simulink model "Simscape_Benchmark_SIM1"  (R2021a)
settings: Solver=ode45  StartTime=0.0  StopTime=PHASE.Ttotal  FixedStep=Benchmark.Sim.Tint  RelTol=1e-5  AbsTol=1e-6
undefined symbols (not defined in the file): Actuators, Analysis, antisym, Benchmark, Bus, Disturbance, FSM, IntialCond, ISOL, K_Coarse_disc_t, Kslew_opt_disc_zoh, Model, MPS, PAYLOAD, PHASE, PMA, RWIsol, RWS, SA, Sensors, Slew, slosh, thr, X, Y, Z
libraries: sm_lib x215, nesl_utility x148, simulink x65, cstblocks x36, sharedtransform x4, vrlib x3, RCTblocks x1
(part 2 of 9)

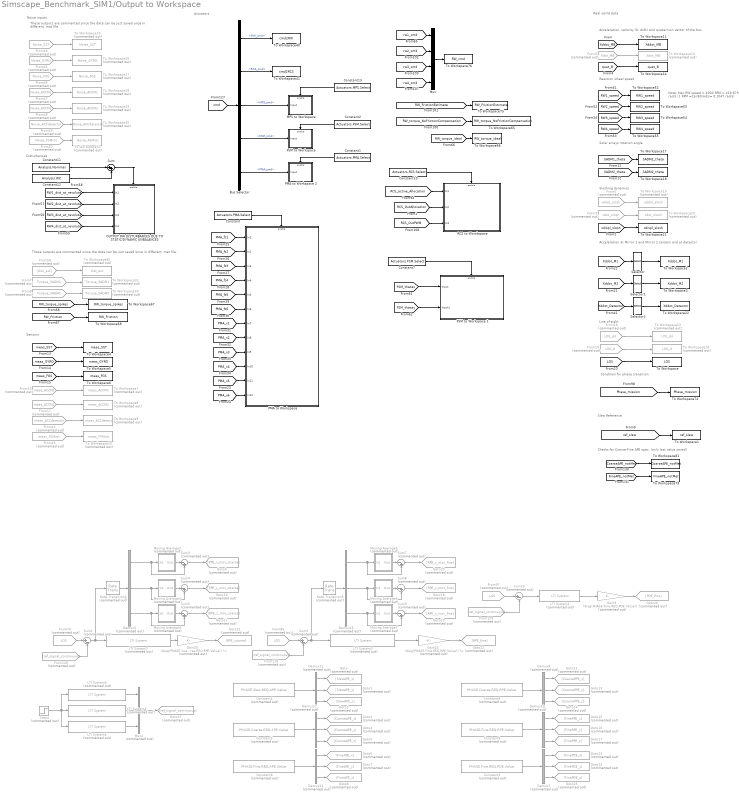
== system Simscape_Benchmark_SIM1/Output to Workspace ==
  note: Note:
      | Max RW speed = 4000 RPM = 418.879 rad/s
      |
      | (1 RPM =2pi/60rad/s= 0.1047 rad/s)
  note: Disturbances
  note: Actuators
  note: Noise inputs
  note: Real world data
  note: Sensors
  note: These outputs are commented since the data can be just saved once in different .mat file.
  note: These outputs are commented since the data can be just saved once in different .mat file.
  note: Acceleration, velocity (6- dofs) and quaternion vector of the bus
  note: Reaction wheel speed
  note: Solar arrays rotation angle
  note: Sloshing dynamics
  note: Acceleration at Mirror 1 and Mirror 2 centers and at detector
  note: Line of sight
  note: Condition for phase transition
  note: Checks for Coarse-Fine APE spec. (only last value saved)
  note: Slew Reference
  Bus Selector : BusSelector  OutputSignals=RW_cmd,RCS_cmd,MPS_cmd,FSM_cmd,PMA_cmd
  Constant : Constant  Value=Actuators.PMA.Select
  Constant1 : Constant  Value=Actuators.PMA.Select
  Constant10 : Constant  Value=Actuators.RCS.Select
  Constant11 : Constant  Value=Analysis.Nominal
  Constant12 : Constant  Value=Analysis.WC
  Constant13 : Constant  Value=Actuators.MPS.Select
  Constant2 : Constant  Value=Actuators.FSM.Select
  Constant3 : Constant  Commented=on  Value=PHASE.Fine.REQ.PDE.Value
  Constant4 : Constant  Commented=on  Value=PHASE.Slew.REQ.APE.Value
  Constant5 : Constant  Commented=on  Value=PHASE.Coarse.REQ.APE.Value
  Constant6 : Constant  Commented=on  Value=PHASE.Fine.REQ.APE.Value
  Constant7 : Constant  Value=Actuators.FSM.Select
  Constant8 : Constant  Commented=on  Value=PHASE.Coarse.REQ.RPE.Value
  Constant9 : Constant  Commented=on  Value=PHASE.Fine.REQ.RPE.Value
  Demux{3,7,9..13,15} (8 alike) : Demux  Commented=on  Outputs=3
  FSM to Workspace : Subsystem  TreatAsAtomicUnit=on
  FSM to Workspace 1 : Subsystem  TreatAsAtomicUnit=on
  From116 : From  Commented=on  GotoTag=ref_signal_continuous
  From120 : From  Commented=on  GotoTag=ref_signal_continuous
  From128 : From  Commented=on  GotoTag=ref_signal_continuous
  From16 : From  Commented=on  GotoTag=meas_ACCM1  TagVisibility=global
  From17 : From  Commented=on  GotoTag=meas_ACCM2  TagVisibility=global
  From18 : From  Commented=on  GotoTag=LOS_dd  TagVisibility=global
  From19 : From  Commented=on  GotoTag=LOS_d  TagVisibility=global
  From3 : From  Commented=on  GotoTag=xdot_slosh  TagVisibility=global
  From42 : From  Commented=on  GotoTag=meas_ACCdetector  TagVisibility=global
  From43 : From  Commented=on  GotoTag=meas_FSMrot  TagVisibility=global
  From44 : From  Commented=on  GotoTag=Noise_SST  TagVisibility=global
  From45 : From  Commented=on  GotoTag=Noise_GYRO  TagVisibility=global
  From46 : From  Commented=on  GotoTag=Noise_FGS  TagVisibility=global
  From47 : From  Commented=on  GotoTag=Noise_ACCM1  TagVisibility=global
  From48 : From  Commented=on  GotoTag=Noise_ACCM2  TagVisibility=global
  From49 : From  Commented=on  GotoTag=Noise_ACCdetector  TagVisibility=global
  From5 : From  Commented=on  GotoTag=xddot_slosh  TagVisibility=global
  From50 : From  Commented=on  GotoTag=Noise_FSMrot  TagVisibility=global
  From59 : From  Commented=on  GotoTag=dist_ext
  From6 : From  Commented=on  GotoTag=Xdot_MB  TagVisibility=global
  From7 : From  Commented=on  GotoTag=Torque_SADM1  TagVisibility=global
  From79 : From  Commented=on  GotoTag=LOS  TagVisibility=global
  From8 : From  Commented=on  GotoTag=Torque_SADM2  TagVisibility=global
  From85 : From  Commented=on  GotoTag=LOS  TagVisibility=global
  From97 : From  Commented=on  GotoTag=LOS  TagVisibility=global
  Gain20 : Gain  Commented=on  Gain=(diag(PHASE.Coarse.REQ.RPE.Value))  Multiplication=Matrix(K*u) (u vector)
  Gain24 : Gain  Commented=on  Gain=(diag(PHASE.Fine.REQ.RPE.Value))  Multiplication=Matrix(K*u) (u vector)
  Gain9 : Gain  Commented=on  Gain=(diag(PHASE.Fine.REQ.PDE.Value))  Multiplication=Matrix(K*u) (u vector)
  Goto : Goto  Commented=on  GotoTag=SlewAPE_x
  Goto1 : Goto  Commented=on  GotoTag=SlewAPE_y
  Goto10 : Goto  Commented=on  GotoTag=RPE_y_mov_coarse
  Goto11 : Goto  Commented=on  GotoTag=RPE_z_mov_coarse
  Goto12 : Goto  Commented=on  GotoTag=CoarseRPE_x
  Goto13 : Goto  Commented=on  GotoTag=CoarseRPE_y
  Goto14 : Goto  Commented=on  GotoTag=CoarseRPE_z
  Goto15 : Goto  Commented=on  GotoTag=FineRPE_x
  Goto16 : Goto  Commented=on  GotoTag=FineRPE_y
  Goto17 : Goto  Commented=on  GotoTag=FineRPE_z
  Goto18 : Goto  Commented=on  GotoTag=RPE_y_mov_fine
  Goto19 : Goto  Commented=on  GotoTag=RPE_z_mov_fine
  Goto2 : Goto  Commented=on  GotoTag=SlewAPE_z
  Goto20 : Goto  Commented=on  GotoTag=RPE_x_mov_fine
  Goto21 : Goto  Commented=on  GotoTag=RPE_coarse
  Goto22 : Goto  Commented=on  GotoTag=RPE_fine
  Goto23 : Goto  Commented=on  GotoTag=FinePDE_x
  Goto24 : Goto  Commented=on  GotoTag=FinePDE_y
  Goto25 : Goto  Commented=on  GotoTag=FinePDE_z
  Goto26 : Goto  Commented=on  GotoTag=PDE_fine
  Goto3 : Goto  Commented=on  GotoTag=CoarseAPE_x
  Goto37 : Goto  Commented=on  GotoTag=ref_signal_continuous
  Goto4 : Goto  Commented=on  GotoTag=CoarseAPE_y
  Goto5 : Goto  Commented=on  GotoTag=CoarseAPE_z
  Goto6 : Goto  Commented=on  GotoTag=FineAPE_x
  Goto7 : Goto  Commented=on  GotoTag=FineAPE_y
  Goto8 : Goto  Commented=on  GotoTag=FineAPE_z
  Goto9 : Goto  Commented=on  GotoTag=RPE_x_mov_coarse
  LTI System1 : cstblocks/LTI System  Commented=on  sys=PHASE.Fine.REQ.PDE.Weight(1:3,1:3)  IC=[]
  LTI System2 : cstblocks/LTI System  Commented=on  sys=PHASE.Coarse.REQ.RPE.Weight(1:3,1:3)  IC=[]
  LTI System3 : cstblocks/LTI System  Commented=on  sys=PHASE.Fine.REQ.RPE.Weight(1:3,1:3)  IC=[]
  LTI System4 : cstblocks/LTI System  Commented=on  sys=Slew.Ref_model.Function_Y  IC=[]
  LTI System5 : cstblocks/LTI System  Commented=on  sys=Slew.Ref_model.Function_Z  IC=[]
  LTI System6 : cstblocks/LTI System  Commented=on  sys=Slew.Ref_model.Function_X  IC=[]
  MPS to Workspace : Subsystem  TreatAsAtomicUnit=on
  Moving Average2 : Subsystem  Description=Replaced Block  Commented=on  InitFcn=error('This block was designed with a newer version of Simulink. Unfortunately, your Simulink version does not support these features.')  mask(Replaced Block){}
      mask help: This block has been replaced with an empty subsystem because it used functionality that is unavailable in Simulink R2021a.
      mask Display: fprintf('Replaced: %s\n','Moving Statistics with Overlap Length not equal to Window Length - 1 (supported from R2022b).')
  Moving Average3 : Subsystem  Description=Replaced Block  Commented=on  InitFcn=error('This block was designed with a newer version of Simulink. Unfortunately, your Simulink version does not support these features.')  mask(Replaced Block){}
      mask help: This block has been replaced with an empty subsystem because it used functionality that is unavailable in Simulink R2021a.
      mask Display: fprintf('Replaced: %s\n','Moving Statistics with Overlap Length not equal to Window Length - 1 (supported from R2022b).')
  Moving Average4 : Subsystem  Description=Replaced Block  Commented=on  InitFcn=error('This block was designed with a newer version of Simulink. Unfortunately, your Simulink version does not support these features.')  mask(Replaced Block){}
      mask help: This block has been replaced with an empty subsystem because it used functionality that is unavailable in Simulink R2021a.
      mask Display: fprintf('Replaced: %s\n','Moving Statistics with Overlap Length not equal to Window Length - 1 (supported from R2022b).')
  Moving Average5 : Subsystem  Description=Replaced Block  Commented=on  InitFcn=error('This block was designed with a newer version of Simulink. Unfortunately, your Simulink version does not support these features.')  mask(Replaced Block){}
      mask help: This block has been replaced with an empty subsystem because it used functionality that is unavailable in Simulink R2021a.
      mask Display: fprintf('Replaced: %s\n','Moving Statistics with Overlap Length not equal to Window Length - 1 (supported from R2022b).')
  Moving Average6 : Subsystem  Description=Replaced Block  Commented=on  InitFcn=error('This block was designed with a newer version of Simulink. Unfortunately, your Simulink version does not support these features.')  mask(Replaced Block){}
      mask help: This block has been replaced with an empty subsystem because it used functionality that is unavailable in Simulink R2021a.
      mask Display: fprintf('Replaced: %s\n','Moving Statistics with Overlap Length not equal to Window Length - 1 (supported from R2022b).')
  Moving Average7 : Subsystem  Description=Replaced Block  Commented=on  InitFcn=error('This block was designed with a newer version of Simulink. Unfortunately, your Simulink version does not support these features.')  mask(Replaced Block){}
      mask help: This block has been replaced with an empty subsystem because it used functionality that is unavailable in Simulink R2021a.
      mask Display: fprintf('Replaced: %s\n','Moving Statistics with Overlap Length not equal to Window Length - 1 (supported from R2022b).')
  Mux : Mux
  Mux4 : Mux  Commented=on  Inputs=3
  OUTPUT RW DISTURBANCES DUE TO STATIC/DYNAMIC UNBALANCES : Subsystem  TreatAsAtomicUnit=on
  PMA to Workspace : Subsystem  TreatAsAtomicUnit=on
  PMA to Workspace 2 : Subsystem  TreatAsAtomicUnit=on
  RCS to Worskspace : Subsystem  TreatAsAtomicUnit=on
  Rate Transition4 : RateTransition  Commented=on  OutPortSampleTime=Model.PayloadMeas_sampling.Ts
  Rate Transition5 : RateTransition  Commented=on  OutPortSampleTime=Model.PayloadMeas_sampling.Ts
  Selector : Selector  InputPortWidth=6  IndexOptions=Index vector (dialog)  Indices=[1 2 3]  OutputSizes=1
  Selector1 : Selector  InputPortWidth=6  IndexOptions=Index vector (dialog)  Indices=[1 2 3]  OutputSizes=1
  Selector2 : Selector  InputPortWidth=6  IndexOptions=Index vector (dialog)  Indices=[1 2 3]  OutputSizes=1
  Step4 : Step  Commented=on  SampleTime=Model.ACS_sampling.Ts
  Sum : Sum  Inputs=|++
  Sum10 : Sum  Commented=on  Inputs=|+-
  Sum2 : Sum  Commented=on  Inputs=|+-
  Sum{3..5,7..9} (6 alike) : Sum  Commented=on  Inputs=|-+
  Sum6 : Sum  Commented=on  Inputs=|+-
  To Workspace : ToWorkspace  VariableName=LOS  SampleTime=Model.PayloadMeas_sampling.Ts
      settings: Save2DSignal=2-D array (concatenate along first dimension)
  To Workspace1 : ToWorkspace  VariableName=ref_slew  SampleTime=Model.PayloadMeas_sampling.Ts
      settings: Save2DSignal=2-D array (concatenate along first dimension)
  To Workspace10 : ToWorkspace  Commented=on  VariableName=meas_FSMrot  SampleTime=-1
      settings: Save2DSignal=2-D array (concatenate along first dimension)
  To Workspace11 : ToWorkspace  VariableName=Xddot_MB  SampleTime=Model.ACS_sampling.Ts
      settings: Save2DSignal=2-D array (concatenate along first dimension)
  To Workspace13 : ToWorkspace  Commented=on  VariableName=Xdot_MB  SampleTime=Model.PayloadMeas_sampling.Ts
      settings: Save2DSignal=2-D array (concatenate along first dimension)
  To Workspace14 : ToWorkspace  VariableName=quat_B  SampleTime=Model.ACS_sampling.Ts
      settings: Save2DSignal=2-D array (concatenate along first dimension)
  To Workspace17 : ToWorkspace  VariableName=SADM1_theta  SampleTime=Model.ACS_sampling.Ts
      settings: Save2DSignal=2-D array (concatenate along first dimension)
  To Workspace18 : ToWorkspace  VariableName=SADM2_theta  SampleTime=Model.ACS_sampling.Ts
      settings: Save2DSignal=2-D array (concatenate along first dimension)
  To Workspace19 : ToWorkspace  Commented=on  VariableName=xddot_slosh  SampleTime=Model.ACS_sampling.Ts
      settings: Save2DSignal=2-D array (concatenate along first dimension)
  To Workspace2 : ToWorkspace  VariableName=Xddot_M1  SampleTime=Model.PayloadMeas_sampling.Ts
      settings: Save2DSignal=2-D array (concatenate along first dimension)
  To Workspace20 : ToWorkspace  Commented=on  VariableName=xdot_slosh  SampleTime=Model.PayloadMeas_sampling.Ts
      settings: Save2DSignal=2-D array (concatenate along first dimension)
  To Workspace21 : ToWorkspace  VariableName=xdispl_slosh  SampleTime=Model.ACS_sampling.Ts
      settings: Save2DSignal=2-D array (concatenate along first dimension)
  To Workspace22 : ToWorkspace  VariableName=Xddot_Detector  SampleTime=Model.PayloadMeas_sampling.Ts
      settings: Save2DSignal=2-D array (concatenate along first dimension)
  To Workspace23 : ToWorkspace  Commented=on  VariableName=LOS_dd  SampleTime=Model.PayloadMeas_sampling.Ts
      settings: Save2DSignal=2-D array (concatenate along first dimension)
  To Workspace24 : ToWorkspace  Commented=on  VariableName=LOS_d  SampleTime=Model.PayloadMeas_sampling.Ts
      settings: Save2DSignal=2-D array (concatenate along first dimension)
  To Workspace25 : ToWorkspace  Commented=on  VariableName=Noise_SST  SampleTime=-1
      settings: Save2DSignal=2-D array (concatenate along first dimension)
  To Workspace26 : ToWorkspace  Commented=on  VariableName=Noise_GYRO  SampleTime=-1
      settings: Save2DSignal=2-D array (concatenate along first dimension)
  To Workspace27 : ToWorkspace  Commented=on  VariableName=Noise_FGS  SampleTime=-1
      settings: Save2DSignal=2-D array (concatenate along first dimension)
  To Workspace28 : ToWorkspace  Commented=on  VariableName=Noise_ACCM1  SampleTime=-1
      settings: Save2DSignal=2-D array (concatenate along first dimension)
  To Workspace29 : ToWorkspace  Commented=on  VariableName=Noise_ACCM2  SampleTime=-1
      settings: Save2DSignal=2-D array (concatenate along first dimension)
  To Workspace3 : ToWorkspace  VariableName=Xddot_M2  SampleTime=Model.PayloadMeas_sampling.Ts
      settings: Save2DSignal=2-D array (concatenate along first dimension)
  To Workspace30 : ToWorkspace  Commented=on  VariableName=Noise_ACCdetector  SampleTime=-1
      settings: Save2DSignal=2-D array (concatenate along first dimension)
  To Workspace31 : ToWorkspace  Commented=on  VariableName=Noise_FSMrot  SampleTime=-1
      settings: Save2DSignal=2-D array (concatenate along first dimension)
  To Workspace32 : ToWorkspace  Commented=on  VariableName=Torque_SADM1  SampleTime=-1
      settings: Save2DSignal=2-D array (concatenate along first dimension)
  To Workspace33 : ToWorkspace  Commented=on  VariableName=Torque_SADM2  SampleTime=-1
      settings: Save2DSignal=2-D array (concatenate along first dimension)
  To Workspace4 : ToWorkspace  VariableName=meas_SST  SampleTime=-1
      settings: Save2DSignal=2-D array (concatenate along first dimension)
  To Workspace40 : ToWorkspace  VariableName=cmd2RW  SampleTime=Model.ACS_sampling.Ts
      settings: Save2DSignal=2-D array (concatenate along first dimension)
  To Workspace41 : ToWorkspace  VariableName=cmd2RCS  SampleTime=Model.ACS_sampling.Ts
      settings: Save2DSignal=2-D array (concatenate along first dimension)
  To Workspace5 : ToWorkspace  VariableName=meas_GYRO  SampleTime=-1
      settings: Save2DSignal=2-D array (concatenate along first dimension)
  To Workspace52 : ToWorkspace  VariableName=RW1_speed  SampleTime=Model.ACS_sampling.Ts
      settings: Save2DSignal=2-D array (concatenate along first dimension)
  To Workspace53 : ToWorkspace  VariableName=RW2_speed  SampleTime=Model.ACS_sampling.Ts
      settings: Save2DSignal=2-D array (concatenate along first dimension)
  To Workspace54 : ToWorkspace  VariableName=RW3_speed  SampleTime=Model.ACS_sampling.Ts
      settings: Save2DSignal=2-D array (concatenate along first dimension)
  To Workspace55 : ToWorkspace  VariableName=RW4_speed  SampleTime=Model.ACS_sampling.Ts
      settings: Save2DSignal=2-D array (concatenate along first dimension)
  To Workspace6 : ToWorkspace  VariableName=meas_FGS  SampleTime=-1
      settings: Save2DSignal=2-D array (concatenate along first dimension)
  To Workspace60 : ToWorkspace  Commented=on  VariableName=dist_ext  SampleTime=-1
      settings: Save2DSignal=2-D array (concatenate along first dimension)
  To Workspace65 : ToWorkspace  VariableName=RW_torque_NoFrictionCompensation  SampleTime=-1
      settings: Save2DSignal=2-D array (concatenate along first dimension)
  To Workspace66 : ToWorkspace  VariableName=RW_torque_ideal  SampleTime=-1
      settings: Save2DSignal=2-D array (concatenate along first dimension)
  To Workspace67 : ToWorkspace  VariableName=RW_torque_spikes  SampleTime=-1
      settings: Save2DSignal=2-D array (concatenate along first dimension)
  To Workspace68 : ToWorkspace  VariableName=RW_Friction  SampleTime=-1
      settings: Save2DSignal=2-D array (concatenate along first dimension)
  To Workspace7 : ToWorkspace  Commented=on  VariableName=meas_ACCM1  SampleTime=-1
      settings: Save2DSignal=2-D array (concatenate along first dimension)
  To Workspace74 : ToWorkspace  VariableName=Phase_mission  SampleTime=-1
      settings: Save2DSignal=2-D array (concatenate along first dimension)
  To Workspace75 : ToWorkspace  VariableName=RW_FrictionEstimate  SampleTime=-1
      settings: Save2DSignal=2-D array (concatenate along first dimension)
  To Workspace76 : ToWorkspace  VariableName=RW_cmd  SampleTime=-1
      settings: Save2DSignal=2-D array (concatenate along first dimension)
  To Workspace79 : ToWorkspace  VariableName=FineAPE_notMet  SampleTime=-1
      settings: MaxDataPoints=1  Save2DSignal=2-D array (concatenate along first dimension)
  To Workspace8 : ToWorkspace  Commented=on  VariableName=meas_ACCM2  SampleTime=-1
      settings: Save2DSignal=2-D array (concatenate along first dimension)
  To Workspace81 : ToWorkspace  VariableName=CoarseAPE_notMet  SampleTime=-1
      settings: MaxDataPoints=1  Save2DSignal=2-D array (concatenate along first dimension)
  To Workspace9 : ToWorkspace  Commented=on  VariableName=meas_ACCdetect  SampleTime=-1
      settings: Save2DSignal=2-D array (concatenate along first dimension)
  wires:
  [meas_SST] -> To Workspace4/1
  [meas_GYRO] -> To Workspace5/1
  [meas_FGS] -> To Workspace6/1
  From16/1 -> To Workspace7/1
  From17/1 -> To Workspace8/1
  From42/1 -> To Workspace9/1
  From43/1 -> To Workspace10/1
  [Xddot_MB] -> To Workspace11/1
  From6/1 -> To Workspace13/1
  [quat_B] -> To Workspace14/1
  [SADM1_theta] -> To Workspace17/1
  [SADM2_theta] -> To Workspace18/1
  From5/1 -> To Workspace19/1
  From3/1 -> To Workspace20/1
  [xdispl_slosh] -> To Workspace21/1
  From44/1 -> To Workspace25/1
  From45/1 -> To Workspace26/1
  From46/1 -> To Workspace27/1
  From47/1 -> To Workspace28/1
  From48/1 -> To Workspace29/1
  From49/1 -> To Workspace30/1
  From50/1 -> To Workspace31/1
  From7/1 -> To Workspace32/1
  From8/1 -> To Workspace33/1
  [RW1_speed] -> To Workspace52/1
  [RW2_speed] -> To Workspace53/1
  [RW3_speed] -> To Workspace54/1
  [RW4_speed] -> To Workspace55/1
  [RW1_dist_at_revolute] -> OUTPUT RW DISTURBANCES DUE TO STATIC/DYNAMIC UNBALANCES/1(In1)
  [RW2_dist_at_revolute] -> OUTPUT RW DISTURBANCES DUE TO STATIC/DYNAMIC UNBALANCES/2(In2)
  [RW3_dist_at_revolute] -> OUTPUT RW DISTURBANCES DUE TO STATIC/DYNAMIC UNBALANCES/3(In3)
  [RW4_dist_at_revolute] -> OUTPUT RW DISTURBANCES DUE TO STATIC/DYNAMIC UNBALANCES/4(In4)
  From59/1 -> To Workspace60/1
  [RW_torque_spikes] -> To Workspace67/1
  [RW_Friction] -> To Workspace68/1
  From18/1 -> To Workspace23/1
  From19/1 -> To Workspace24/1
  [LOS] -> To Workspace/1
  [Xddot_M1] -> Selector/1
  [Xddot_M2] -> Selector1/1
  [Xddot_Detector] -> Selector2/1
  Constant4/1 -> Demux11/1
  Constant5/1 -> Demux12/1
  Constant6/1 -> Demux13/1
  Demux11/1 -> Goto/1
  Demux11/2 -> Goto1/1
  Demux11/3 -> Goto2/1
  Demux12/1 -> Goto3/1
  Demux12/2 -> Goto4/1
  Demux12/3 -> Goto5/1
  Demux13/3 -> Goto8/1
  Demux13/2 -> Goto7/1
  Demux13/1 -> Goto6/1
  From79/1 -> Sum2/1
  Demux10/2 -> Goto16/1
  Constant8/1 -> Demux9/1
  Demux10/1 -> Goto15/1
  Demux9/2 -> Goto13/1
  Demux9/3 -> Goto14/1
  Constant9/1 -> Demux10/1
  Demux9/1 -> Goto12/1
  Demux10/3 -> Goto17/1
  LTI System2/1 -> Gain20/1
  Gain20/1 -> Goto21/1
  Demux3/1 -> Sum3/2, Moving Average2/1(In1)
  Moving Average2/1(Out1) -> Sum3/1
  Rate Transition4/1 -> Demux3/1
  Sum2/1 -> LTI System2/1, Rate Transition4/1
  Demux3/2 -> Sum4/2, Moving Average3/1(In1)
  Moving Average3/1(Out1) -> Sum4/1
  Demux3/3 -> Sum5/2, Moving Average4/1(In1)
  Moving Average4/1(Out1) -> Sum5/1
  Sum3/1 -> Goto9/1
  Sum4/1 -> Goto10/1
  Sum5/1 -> Goto11/1
  Demux15/2 -> Sum8/2, Moving Average6/1(In1)
  Sum6/1 -> LTI System3/1, Rate Transition5/1
  Rate Transition5/1 -> Demux15/1
  Moving Average5/1(Out1) -> Sum7/1
  Demux15/1 -> Sum7/2, Moving Average5/1(In1)
  LTI System3/1 -> Gain24/1
  Demux15/3 -> Sum9/2, Moving Average7/1(In1)
  Sum7/1 -> Goto20/1
  Moving Average7/1(Out1) -> Sum9/1
  From85/1 -> Sum6/1
  Sum9/1 -> Goto19/1
  Sum8/1 -> Goto18/1
  Moving Average6/1(Out1) -> Sum8/1
  Gain24/1 -> Goto22/1
  From97/1 -> Sum10/1
  Sum10/1 -> LTI System1/1
  Gain9/1 -> Goto26/1
  LTI System1/1 -> Gain9/1
  Demux7/3 -> Goto25/1
  Constant3/1 -> Demux7/1
  Demux7/2 -> Goto24/1
  Demux7/1 -> Goto23/1
  [Phase_mission] -> To Workspace74/1
  [RW_torque_NoFrictionCompensation] -> To Workspace65/1
  [RW_torque_ideal] -> To Workspace66/1
  [RW_FrictionEstimate] -> To Workspace75/1
  [rw1_cmd] -> Mux/1
  [rw2_cmd] -> Mux/2
  [rw4_cmd] -> Mux/4
  [rw3_cmd] -> Mux/3
  Mux/1 -> To Workspace76/1
  [cmd] -> Bus Selector/1
  Mux4/1 -> Goto37/1
  LTI System5/1 -> Mux4/3
  LTI System4/1 -> Mux4/2
  Step4/1 -> LTI System5/1, LTI System6/1, LTI System4/1
  LTI System6/1 -> Mux4/1
  From116/1 -> Sum6/2
  From120/1 -> Sum10/2
  From128/1 -> Sum2/2
  [FineAPE_notMet] -> To Workspace79/1
  [CoarseAPE_notMet] -> To Workspace81/1
  Bus Selector/1 -> To Workspace40/1  "<RW_cmd>"
  Bus Selector/2 -> To Workspace41/1  "<RCS_cmd>"
  Bus Selector/3 -> MPS to Workspace/1(Input)  "<MPS_cmd>"
  Bus Selector/4 -> FSM to Workspace/1(Input)  "<FSM_cmd>"
  Bus Selector/5 -> PMA to Workspace 2/1(Input)  "<PMA_cmd>"
  Constant1/1 -> PMA to Workspace 2/Enable
  Constant2/1 -> FSM to Workspace/Enable
  Constant7/1 -> FSM to Workspace 1/Enable
  Constant10/1 -> RCS to Worskspace/Enable
  [FSM_thetax] -> FSM to Workspace 1/1(Input)
  [FSM_thetay] -> FSM to Workspace 1/2(Input1)
  Constant/1 -> PMA to Workspace/Enable
  [PMA_fz1] -> PMA to Workspace/1(In1)
  [PMA_fz2] -> PMA to Workspace/2(In2)
  [PMA_fz3] -> PMA to Workspace/3(In3)
  [PMA_fz4] -> PMA to Workspace/4(In4)
  [PMA_fz5] -> PMA to Workspace/5(In5)
  [PMA_fz6] -> PMA to Workspace/6(In6)
  [PMA_x1] -> PMA to Workspace/7(In7)
  [PMA_x2] -> PMA to Workspace/8(In8)
  [PMA_x3] -> PMA to Workspace/9(In9)
  [PMA_x4] -> PMA to Workspace/10(In10)
  [PMA_x5] -> PMA to Workspace/11(In11)
  [PMA_x6] -> PMA to Workspace/12(In12)
  [RCS_active_Allocation] -> RCS to Worskspace/1(In1)
  [RCS_OutAllocation] -> RCS to Worskspace/2(In2)
  [RCS_OutPWM] -> RCS to Worskspace/3(In3)
  Constant11/1 -> Sum/1
  Sum/1 -> OUTPUT RW DISTURBANCES DUE TO STATIC/DYNAMIC UNBALANCES/Enable
  Constant12/1 -> Sum/2
  Selector/1 -> To Workspace2/1
  Selector1/1 -> To Workspace3/1
  Selector2/1 -> To Workspace22/1
  Constant13/1 -> MPS to Workspace/Enable
  [ref_slew] -> To Workspace1/1

== system Simscape_Benchmark_SIM1/RW broadband disturbance ==
  note: Disturbance.RW.BroadBand.SampleTime=0.005;
      | Disturbance.RW.BroadBand.Mean=0;
      | sigmaF=5e-4;
      | sigmaT=1e-4;
      | Disturbance.RW.BroadBand.RW1Fxy = (sigmaF*sqrt(Disturbance.RW.BroadBand.SampleTime))^2;
      | Disturbance.RW.BroadBand.RW1Txy = (sigmaT*sqrt(Disturbance.RW.BroadBand.SampleTime))^2;
      | Disturbance.RW.BroadBand.RW1_Seed = [2111,2112,2113,2114];
  Band-Limited White Noise1 : simulink/Sources/Band-Limited White Noise  Cov=Disturbance.RW.BroadBand.RW2Fxy  Ts=Disturbance.RW.BroadBand.SampleTime  seed=Disturbance.RW.BroadBand.RW2_Seed(1)
  Band-Limited White Noise10 : simulink/Sources/Band-Limited White Noise  Cov=Disturbance.RW.BroadBand.RW4Fxy  Ts=Disturbance.RW.BroadBand.SampleTime  seed=Disturbance.RW.BroadBand.RW4_Seed(2)
  Band-Limited White Noise11 : simulink/Sources/Band-Limited White Noise  Cov=Disturbance.RW.BroadBand.RW1Fxy  Ts=Disturbance.RW.BroadBand.SampleTime  seed=Disturbance.RW.BroadBand.RW1_Seed(1)
  Band-Limited White Noise12 : simulink/Sources/Band-Limited White Noise  Cov=Disturbance.RW.BroadBand.RW1Fxy  Ts=Disturbance.RW.BroadBand.SampleTime  seed=Disturbance.RW.BroadBand.RW1_Seed(2)
  Band-Limited White Noise13 : simulink/Sources/Band-Limited White Noise  Cov=Disturbance.RW.BroadBand.RW1Txy  Ts=Disturbance.RW.BroadBand.SampleTime  seed=Disturbance.RW.BroadBand.RW1_Seed(3)
  Band-Limited White Noise14 : simulink/Sources/Band-Limited White Noise  Cov=Disturbance.RW.BroadBand.RW1Txy  Ts=Disturbance.RW.BroadBand.SampleTime  seed=Disturbance.RW.BroadBand.RW1_Seed(4)
  Band-Limited White Noise15 : simulink/Sources/Band-Limited White Noise  Cov=Disturbance.RW.BroadBand.RW4Txy  Ts=Disturbance.RW.BroadBand.SampleTime  seed=Disturbance.RW.BroadBand.RW4_Seed(3)
  Band-Limited White Noise16 : simulink/Sources/Band-Limited White Noise  Cov=Disturbance.RW.BroadBand.RW4Txy  Ts=Disturbance.RW.BroadBand.SampleTime  seed=Disturbance.RW.BroadBand.RW4_Seed(4)
  Band-Limited White Noise2 : simulink/Sources/Band-Limited White Noise  Cov=Disturbance.RW.BroadBand.RW2Fxy  Ts=Disturbance.RW.BroadBand.SampleTime  seed=Disturbance.RW.BroadBand.RW2_Seed(2)
  Band-Limited White Noise3 : simulink/Sources/Band-Limited White Noise  Cov=Disturbance.RW.BroadBand.RW2Txy  Ts=Disturbance.RW.BroadBand.SampleTime  seed=Disturbance.RW.BroadBand.RW2_Seed(3)
  Band-Limited White Noise4 : simulink/Sources/Band-Limited White Noise  Cov=Disturbance.RW.BroadBand.RW2Txy  Ts=Disturbance.RW.BroadBand.SampleTime  seed=Disturbance.RW.BroadBand.RW2_Seed(4)
  Band-Limited White Noise5 : simulink/Sources/Band-Limited White Noise  Cov=Disturbance.RW.BroadBand.RW3Fxy  Ts=Disturbance.RW.BroadBand.SampleTime  seed=Disturbance.RW.BroadBand.RW1_Seed(1)
  Band-Limited White Noise6 : simulink/Sources/Band-Limited White Noise  Cov=Disturbance.RW.BroadBand.RW3Fxy  Ts=Disturbance.RW.BroadBand.SampleTime  seed=Disturbance.RW.BroadBand.RW1_Seed(2)
  Band-Limited White Noise7 : simulink/Sources/Band-Limited White Noise  Cov=Disturbance.RW.BroadBand.RW3Txy  Ts=Disturbance.RW.BroadBand.SampleTime  seed=Disturbance.RW.BroadBand.RW1_Seed(3)
  Band-Limited White Noise8 : simulink/Sources/Band-Limited White Noise  Cov=Disturbance.RW.BroadBand.RW3Txy  Ts=Disturbance.RW.BroadBand.SampleTime  seed=Disturbance.RW.BroadBand.RW1_Seed(4)
  Band-Limited White Noise9 : simulink/Sources/Band-Limited White Noise  Cov=Disturbance.RW.BroadBand.RW4Fxy  Ts=Disturbance.RW.BroadBand.SampleTime  seed=Disturbance.RW.BroadBand.RW4_Seed(1)
  Disturbance.RW.BroadBand.SelectSim : Gain  Gain=Disturbance.RW.BroadBand.SelectSim
  Ground{1..4} (4 alike) : Ground
  Mux : Mux
  Mux{1..4} (4 alike) : Mux  Inputs=[1,1,1,1,1]
  RWdist : Outport
  wires:
  Ground3/1 -> Mux1/3
  Mux1/1 -> Mux/1
  Band-Limited White Noise12/1 -> Mux1/2
  Band-Limited White Noise11/1 -> Mux1/1
  Band-Limited White Noise13/1 -> Mux1/4
  Band-Limited White Noise14/1 -> Mux1/5
  Ground1/1 -> Mux2/3
  Band-Limited White Noise3/1 -> Mux2/4
  Band-Limited White Noise4/1 -> Mux2/5
  Mux2/1 -> Mux/2
  Band-Limited White Noise1/1 -> Mux2/1
  Band-Limited White Noise2/1 -> Mux2/2
  Disturbance.RW.BroadBand.SelectSim/1 -> RWdist/1
  Mux3/1 -> Mux/3
  Band-Limited White Noise5/1 -> Mux3/1
  Band-Limited White Noise8/1 -> Mux3/5
  Band-Limited White Noise7/1 -> Mux3/4
  Ground2/1 -> Mux3/3
  Band-Limited White Noise6/1 -> Mux3/2
  Mux4/1 -> Mux/4
  Band-Limited White Noise9/1 -> Mux4/1
  Band-Limited White Noise16/1 -> Mux4/5
  Band-Limited White Noise15/1 -> Mux4/4
  Ground4/1 -> Mux4/3
  Band-Limited White Noise10/1 -> Mux4/2
  Mux/1 -> Disturbance.RW.BroadBand.SelectSim/1

== system Simscape_Benchmark_SIM1/SADM disturbance ==
  Constant : Constant  Value=0.5
  Constant1 : Constant  Value=0.5
  Disturbance.SADM.BroadBand.SelectSim : Gain  Gain=Disturbance.SADM.BroadBand.SelectSim
  Disturbance.SADM.BroadBand.SelectSim 2 : Gain  Gain=Disturbance.SADM.BroadBand.SelectSim
  Disturbance.SADM.SelectSim : Gain  Gain=Disturbance.SADM.SelectSim
  Disturbance.SADM.SelectSim 2 : Gain  Gain=Disturbance.SADM.SelectSim
  Random Number : RandomNumber  Mean=Disturbance.SADM.BroadBand.Mean  Variance=Disturbance.SADM.BroadBand.Variance  Seed=Disturbance.SADM.BroadBand.Seed1  SampleTime=Disturbance.SADM.BroadBand.SampleTime
  Random Number1 : RandomNumber  Mean=Disturbance.SADM.BroadBand.Mean  Variance=Disturbance.SADM.BroadBand.Variance  Seed=Disturbance.SADM.BroadBand.Seed2  SampleTime=Disturbance.SADM.BroadBand.SampleTime
  Sawtooth Generator1 : SignalGenerator  WaveForm=sawtooth  Amplitude=Disturbance.SADM.Amplitude2  Frequency=Disturbance.SADM.sawtooth.omega  Units=rad/sec
  Sawtooth Generator2 : SignalGenerator  WaveForm=sawtooth  Amplitude=Disturbance.SADM.Amplitude1  Frequency=Disturbance.SADM.sawtooth.omega  Units=rad/sec
  Sum : Sum  Inputs=|++
  Sum1 : Sum  Inputs=|++
  Sum2 : Sum  Inputs=|+-
  Sum3 : Sum  Inputs=|+-
  Torque_SADM1 : Outport
  Torque_SADM2 : Outport  Port=2
  wires:
  Sum2/1 -> Disturbance.SADM.SelectSim/1
  Sum3/1 -> Disturbance.SADM.SelectSim 2/1
  Disturbance.SADM.SelectSim/1 -> Sum/1
  Disturbance.SADM.SelectSim 2/1 -> Sum1/1
  Sum/1 -> Torque_SADM1/1
  Random Number/1 -> Disturbance.SADM.BroadBand.SelectSim/1
  Sum1/1 -> Torque_SADM2/1
  Random Number1/1 -> Disturbance.SADM.BroadBand.SelectSim 2/1
  Disturbance.SADM.BroadBand.SelectSim/1 -> Sum/2
  Disturbance.SADM.BroadBand.SelectSim 2/1 -> Sum1/2
  Sawtooth Generator2/1 -> Sum2/1
  Constant/1 -> Sum2/2
  Sawtooth Generator1/1 -> Sum3/1
  Constant1/1 -> Sum3/2

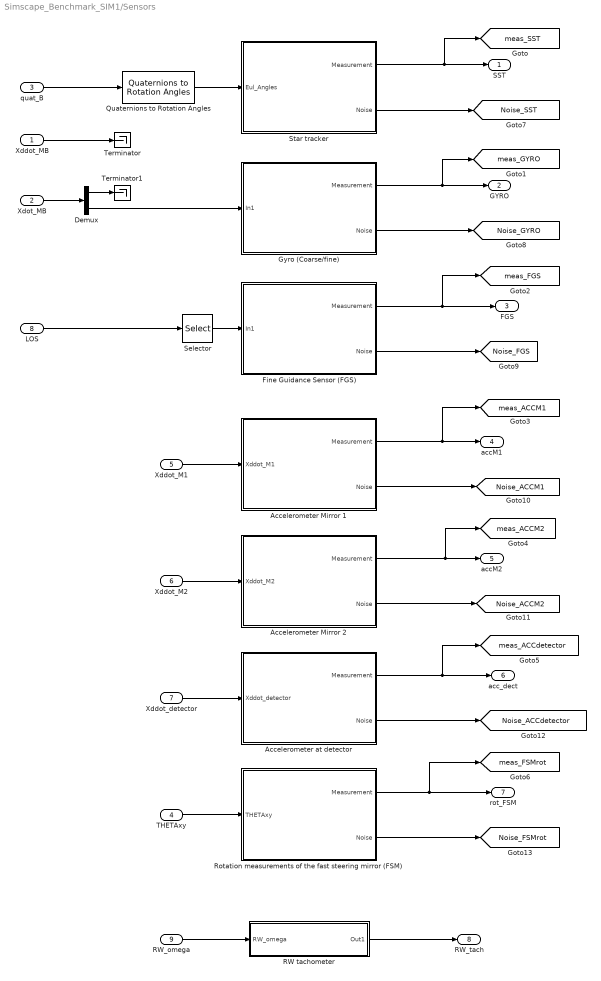
== system Simscape_Benchmark_SIM1/Sensors ==
  Xddot_MB : Inport
  Xdot_MB : Inport  Port=2
  quat_B : Inport  Port=3
  THETAxy : Inport  Port=4
  Xddot_M1 : Inport  Port=5
  Xddot_M2 : Inport  Port=6
  Xddot_detector : Inport  Port=7
  LOS : Inport  Port=8
  RW_omega : Inport  Port=9
  Accelerometer Mirror 1 : Subsystem
  Accelerometer Mirror 2 : Subsystem
  Accelerometer at detector : Subsystem
  Demux : Demux  Outputs=[3,3]
  Fine Guidance Sensor (FGS) : Subsystem
  Gyro (Coarse/fine) : Subsystem
  Quaternions to Rotation Angles : sharedtransform/Quaternions to Rotation Angles  rotationOrder=XYZ  aMode=aMode
      settings: SourceProductBaseCode=AE,PW,DR,MT,UV,VE
  RW tachometer : Subsystem
  Rotation measurements of the fast steering mirror (FSM) : Subsystem
  Selector : Selector  InputPortWidth=3  IndexOptions=Index vector (dialog)  Indices=[1 2]  OutputSizes=1
  Star tracker : Subsystem
  Terminator : Terminator
  Terminator1 : Terminator
  SST : Outport
  GYRO : Outport  Port=2
  FGS : Outport  Port=3
  accM1 : Outport  Port=4
  accM2 : Outport  Port=5
  acc_dect : Outport  Port=6
  rot_FSM : Outport  Port=7
  RW_tach : Outport  Port=8
  tag scope: Noise_ACCM1=global, Noise_ACCM2=global, Noise_ACCdetector=global, Noise_FGS=global, Noise_FSMrot=global, Noise_GYRO=global, Noise_SST=global, meas_ACCM1=global, meas_ACCM2=global, meas_ACCdetector=global, meas_FGS=global, meas_FSMrot=global, meas_GYRO=global, meas_SST=global
  wires:
  Star tracker/1(Measurement) -> [meas_SST], SST/1
  Gyro (Coarse/fine)/1(Measurement) -> [meas_GYRO], GYRO/1
  Fine Guidance Sensor (FGS)/1(Measurement) -> [meas_FGS], FGS/1
  Accelerometer Mirror 1/1(Measurement) -> accM1/1, [meas_ACCM1]
  Accelerometer Mirror 2/1(Measurement) -> [meas_ACCM2], accM2/1
  Accelerometer at detector/1(Measurement) -> [meas_ACCdetector], acc_dect/1
  Rotation measurements of the fast steering mirror (FSM)/1(Measurement) -> rot_FSM/1, [meas_FSMrot]
  Xdot_MB/1 -> Demux/1
  Demux/2 -> Gyro (Coarse/fine)/1(In1)
  Demux/1 -> Terminator1/1
  quat_B/1 -> Quaternions to Rotation Angles/1
  Star tracker/2(Noise) -> [Noise_SST]
  Gyro (Coarse/fine)/2(Noise) -> [Noise_GYRO]
  Fine Guidance Sensor (FGS)/2(Noise) -> [Noise_FGS]
  Accelerometer Mirror 1/2(Noise) -> [Noise_ACCM1]
  Accelerometer Mirror 2/2(Noise) -> [Noise_ACCM2]
  Accelerometer at detector/2(Noise) -> [Noise_ACCdetector]
  Rotation measurements of the fast steering mirror (FSM)/2(Noise) -> [Noise_FSMrot]
  Xddot_M1/1 -> Accelerometer Mirror 1/1(Xddot_M1)
  Xddot_detector/1 -> Accelerometer at detector/1(Xddot_detector)
  Xddot_M2/1 -> Accelerometer Mirror 2/1(Xddot_M2)
  THETAxy/1 -> Rotation measurements of the fast steering mirror (FSM)/1(THETAxy)
  Selector/1 -> Fine Guidance Sensor (FGS)/1(In1)
  LOS/1 -> Selector/1
  Quaternions to Rotation Angles/1 -> Star tracker/1(Eul_Angles)
  Xddot_MB/1 -> Terminator/1
  RW tachometer/1(Out1) -> RW_tach/1
  RW_omega/1 -> RW tachometer/1(RW_omega)

== system Simscape_Benchmark_SIM1/Controllers/Coarse 2 fine  ==
  note: 20 s
  note: Select from the " bus selector" block the outputs from the "meas" signal that the user uses as input of the controller
  note: This part can be modified by the user by selecting which measurements to use and the controller to be implemented.
  note: This part can be modified by the user by selecting which strategy to implement for the switching between two controllers
  note: REMARK: Leave the name of the signals in the lines entering and exiting the "bus creator" block unaltered.
  note: 4 s
  meas : Inport
  ref : Inport  Port=2
  TransitionCoarse2FineActivation : Inport  Port=3
  Activation of fine controller : MATLAB Function  TreatAsAtomicUnit=on  SystemSampleTime=Model.PayloadMeas_sampling.Ts
  Bus Creator : BusCreator  Inputs=5
  Bus Selector2 : BusSelector  OutputSignals=FGS_meas,AccM1_meas,AccM2_meas,Accdect_meas,rotFSM_meas
  Bus Selector3 : BusSelector  OutputSignals=SST_meas,GYRO_meas
  Constant16 : Constant  Value=Model.PayloadMeas_sampling.Ts
  Constant20 : Constant  Value=zeros(6,1)  SampleTime=Model.PayloadMeas_sampling.Ts
  Constant21 : Constant  Value=zeros(3,1)  SampleTime=Model.MPS_sampling.Ts
  Constant22 : Constant  Value=zeros(3,1)  SampleTime=Model.ACS_sampling.Ts
  Demux1 : Demux  Outputs=3
  Demux2 : Demux  Outputs=3
  Demux3 : Demux  Outputs=3
  Discrete State-Space1 : DiscreteStateSpace  A=K_Coarse_disc_t.A  B=K_Coarse_disc_t.B  C=K_Coarse_disc_t.C  D=K_Coarse_disc_t.D  SampleTime=Model.ACS_sampling.Ts
  Gain{1..4} (4 alike) : Gain
  LTI System : cstblocks/LTI System  sys=K_FSM_disc_t  IC=[]
  LTI System1 : cstblocks/LTI System  sys=W_lowPass_activation_d  IC=[]
  Mux2 : Mux  Inputs=5
  Mux3 : Mux  Inputs=6
  Product : Product
  Selector : Selector  InputPortWidth=3  IndexOptions=Index vector (dialog)  Indices=[1 2]  OutputSizes=1
  Selector1 : Selector  InputPortWidth=6  IndexOptions=Index vector (dialog)  Indices=[1,2,4,5]  OutputSizes=1
  Selector2 : Selector  InputPortWidth=6  IndexOptions=Index vector (dialog)  Indices=[1,2,4,5]  OutputSizes=1
  Slope : Constant  Value=0.05
  Slope1 : Constant  Commented=on  Value=0.25
  Sum : Sum  Inputs=-+
  Sum1 : Sum  Inputs=+-
  Sum2 : Sum  Inputs=+-
  Sum6 : Sum  Inputs=+-
  cmd : Outport
  wires:
  Bus Creator/1 -> cmd/1  "cmd"
  Constant22/1 -> Bus Creator/2  "RCS_cmd"
  Constant20/1 -> Bus Creator/5  "PMA_cmd"
  Discrete State-Space1/1 -> Bus Creator/1  "RW_cmd"
  Constant21/1 -> Bus Creator/3  "MPS_cmd"
  Mux2/1 -> LTI System/1
  Bus Selector2/3 -> Selector2/1  "<AccM2_meas>"
  Bus Selector2/2 -> Selector1/1  "<AccM1_meas>"
  Bus Selector2/4 -> Gain3/1  "<Accdect_meas>"
  Bus Selector2/5 -> Gain4/1  "<rotFSM_meas>"
  LTI System/1 -> Product/1  "FSM_cmd"
  Demux1/1 -> Sum6/2
  Demux1/3 -> Sum2/2
  Bus Selector3/2 -> Demux3/1  "<GYRO_meas>"
  Demux2/3 -> Sum2/1
  Sum2/1 -> Mux3/5
  Bus Selector3/1 -> Demux2/1  "<SST_meas>"
  Demux1/2 -> Sum1/2
  Sum1/1 -> Mux3/3
  meas/1 -> Bus Selector2/1, Bus Selector3/1
  Demux3/2 -> Mux3/4
  Mux3/1 -> Discrete State-Space1/1
  Demux2/2 -> Sum1/1
  Sum6/1 -> Mux3/1
  Demux2/1 -> Sum6/1
  Demux3/1 -> Mux3/2
  Demux3/3 -> Mux3/6
  Product/1 -> Bus Creator/4  "FSM_cmd"
  Constant16/1 -> Activation of fine controller/2(sampling)
  Slope/1 -> Activation of fine controller/3(Slope)
  Activation of fine controller/1(out) -> LTI System1/1
  Selector/1 -> Sum/1
  Bus Selector2/1 -> Sum/2  "<FGS_meas>"
  Sum/1 -> Mux2/5
  Gain2/1 -> Mux2/1
  Gain1/1 -> Mux2/2
  Gain3/1 -> Mux2/3
  Gain4/1 -> Mux2/4
  ref/1 -> Selector/1, Demux1/1
  TransitionCoarse2FineActivation/1 -> Activation of fine controller/1(TransitionCoarse2FineActivation)
  Selector1/1 -> Gain2/1
  Selector2/1 -> Gain1/1
  LTI System1/1 -> Product/2

== system Simscape_Benchmark_SIM1/Controllers/Coarse pointing ==
  note: This part can be modified by the user by selecting which measurements to use and the comtroller to be implemented.
  note: REMARK: Leave the name of the signals in the lines entering and exiting the "bus creator" block unaltered.
  note: Select from the " bus selector" block the outputs from the "meas" signal that the user uses as input of the controller
  meas : Inport
  ref : Inport  Port=2
  Bus Creator : BusCreator  Inputs=5
  Bus Selector1 : BusSelector  OutputSignals=SST_meas,GYRO_meas
  Constant25 : Constant  Value=zeros(6,1)  SampleTime=Model.PayloadMeas_sampling.Ts
  Constant26 : Constant  Value=zeros(2,1)  SampleTime=Model.PayloadMeas_sampling.Ts
  Constant27 : Constant  Value=zeros(3,1)  SampleTime=Model.MPS_sampling.Ts
  Constant28 : Constant  Value=zeros(3,1)  SampleTime=Model.ACS_sampling.Ts
  Demux1 : Demux  Outputs=3
  Demux10 : Demux  Outputs=3
  Demux9 : Demux  Outputs=3
  Discrete State-Space1 : DiscreteStateSpace  A=K_Coarse_disc_t.A  B=K_Coarse_disc_t.B  C=K_Coarse_disc_t.C  D=K_Coarse_disc_t.D  SampleTime=Model.ACS_sampling.Ts
  Mux2 : Mux  Inputs=6
  Sum1 : Sum  Inputs=+-
  Sum2 : Sum  Inputs=+-
  Sum6 : Sum  Inputs=+-
  <cmd> : Outport
  wires:
  Demux9/3 -> Mux2/6
  Demux10/1 -> Sum6/1
  Constant25/1 -> Bus Creator/5  "PMA_cmd"
  Constant27/1 -> Bus Creator/3  "MPS_cmd"
  Demux9/2 -> Mux2/4
  Constant28/1 -> Bus Creator/2  "RCS_cmd"
  Bus Selector1/2 -> Demux9/1  "<GYRO_meas>"
  Demux10/2 -> Sum1/1
  Demux9/1 -> Mux2/2
  Mux2/1 -> Discrete State-Space1/1
  Constant26/1 -> Bus Creator/4  "FSM_cmd"
  Discrete State-Space1/1 -> Bus Creator/1  "RW_cmd"
  Bus Creator/1 -> <cmd>/1  "cmd"
  Bus Selector1/1 -> Demux10/1  "<SST_meas>"
  meas/1 -> Bus Selector1/1
  ref/1 -> Demux1/1
  Demux1/1 -> Sum6/2
  Sum6/1 -> Mux2/1
  Demux1/2 -> Sum1/2
  Sum1/1 -> Mux2/3
  Demux10/3 -> Sum2/1
  Demux1/3 -> Sum2/2
  Sum2/1 -> Mux2/5

== system Simscape_Benchmark_SIM1/Controllers/Fine pointing ==
  note: REMARK: Leave the name of the signals in the lines entering and exiting the "bus creator" block unaltered.
  note: Select from the " bus selector" block the outputs from the "meas" signal that the user uses as input of the controller
  note: This part can be modified by the user by selecting which measurements to use and the controller to be implemented.
  meas : Inport
  Input : Inport  Port=2
  Bus Creator : BusCreator  Inputs=5
  Bus Selector2 : BusSelector  OutputSignals=FGS_meas,AccM1_meas,AccM2_meas,Accdect_meas,rotFSM_meas
  Bus Selector3 : BusSelector  OutputSignals=SST_meas,GYRO_meas
  Constant20 : Constant  Value=zeros(6,1)  SampleTime=Model.PayloadMeas_sampling.Ts
  Constant21 : Constant  Value=zeros(3,1)  SampleTime=Model.MPS_sampling.Ts
  Constant22 : Constant  Value=zeros(3,1)  SampleTime=Model.ACS_sampling.Ts
  Demux1 : Demux  Outputs=3
  Demux2 : Demux  Outputs=3
  Demux3 : Demux  Outputs=3
  Discrete State-Space1 : DiscreteStateSpace  A=K_Coarse_disc_t.A  B=K_Coarse_disc_t.B  C=K_Coarse_disc_t.C  D=K_Coarse_disc_t.D  SampleTime=Model.ACS_sampling.Ts
  Gain : Gain  Gain=0
  Gain1 : Gain  Gain=0
  Gain2 : Gain  Gain=0
  Gain3 : Gain
  LTI System : cstblocks/LTI System  sys=K_FSM_disc_t  IC=[]
  Mux2 : Mux  Inputs=5
  Mux3 : Mux  Inputs=6
  Selector : Selector  InputPortWidth=3  IndexOptions=Index vector (dialog)  Indices=[1 2]  OutputSizes=1
  Selector1 : Selector  InputPortWidth=6  IndexOptions=Index vector (dialog)  Indices=[1,2,4,5]  OutputSizes=1
  Selector2 : Selector  InputPortWidth=6  IndexOptions=Index vector (dialog)  Indices=[1,2,4,5]  OutputSizes=1
  Sum : Sum  Inputs=-+
  Sum1 : Sum  Inputs=+-
  Sum2 : Sum  Inputs=+-
  Sum6 : Sum  Inputs=+-
  cmd : Outport
  wires:
  Sum/1 -> Mux2/5
  Bus Selector2/4 -> Gain2/1  "<Accdect_meas>"
  Bus Selector2/5 -> Gain3/1  "<rotFSM_meas>"
  Bus Selector2/3 -> Selector2/1  "<AccM2_meas>"
  Mux2/1 -> LTI System/1
  Bus Selector2/1 -> Sum/2  "<FGS_meas>"
  Demux3/3 -> Mux3/6
  Demux2/1 -> Sum6/1
  Demux2/2 -> Sum1/1
  Sum6/1 -> Mux3/1
  Demux3/1 -> Mux3/2
  Sum1/1 -> Mux3/3
  Demux2/3 -> Sum2/1
  Demux1/2 -> Sum1/2
  Sum2/1 -> Mux3/5
  Bus Selector3/2 -> Demux3/1  "<GYRO_meas>"
  Demux1/3 -> Sum2/2
  Demux1/1 -> Sum6/2
  Bus Selector2/2 -> Selector1/1  "<AccM1_meas>"
  Bus Selector3/1 -> Demux2/1  "<SST_meas>"
  LTI System/1 -> Bus Creator/4  "FSM_cmd"
  Constant22/1 -> Bus Creator/2  "RCS_cmd"
  Selector/1 -> Sum/1
  Constant21/1 -> Bus Creator/3  "MPS_cmd"
  Mux3/1 -> Discrete State-Space1/1
  Demux3/2 -> Mux3/4
  meas/1 -> Bus Selector2/1, Bus Selector3/1
  Bus Creator/1 -> cmd/1  "cmd"
  Constant20/1 -> Bus Creator/5  "PMA_cmd"
  Discrete State-Space1/1 -> Bus Creator/1  "RW_cmd"
  Gain/1 -> Mux2/1
  Gain1/1 -> Mux2/2
  Gain2/1 -> Mux2/3
  Gain3/1 -> Mux2/4
  Input/1 -> Selector/1, Demux1/1
  Selector1/1 -> Gain/1
  Selector2/1 -> Gain1/1

== system Simscape_Benchmark_SIM1/Controllers/Slew ==
  note: REMARK: Leave the name of the signals in the lines entering and exiting the "bus creator" block unaltered.
  note: This part can be modified by the user by selecting which measurements to use and the controller to be implemented.
  note: REMARK: Leave the name of the signals in the lines entering and exiting the "bus creator" block unaltered.
  note: Select from the " bus selector" block the outputs from the "meas" signal that the user uses as input of the controller
  meas : Inport
  ref : Inport  Port=2
  slew_deactivation : Inport  Port=3
  Bus Creator : BusCreator  Inputs=5
  Bus Creator2 : BusCreator  Inputs=5
  Bus Selector1 : BusSelector  OutputSignals=SST_meas,GYRO_meas
  Constant : Constant  Value=zeros(3,1)  SampleTime=Model.ACS_sampling.Ts
  Constant20 : Constant  Value=zeros(6,1)  SampleTime=Model.PayloadMeas_sampling.Ts
  Constant21 : Constant  Value=zeros(2,1)  SampleTime=Model.PayloadMeas_sampling.Ts
  Constant22 : Constant  Value=zeros(3,1)  SampleTime=Model.MPS_sampling.Ts
  Constant23 : Constant  Value=zeros(3,1)  SampleTime=Model.ACS_sampling.Ts
  Constant24 : Constant  Value=zeros(3,1)  SampleTime=Model.ACS_sampling.Ts
  Constant25 : Constant  Value=zeros(6,1)  SampleTime=Model.PayloadMeas_sampling.Ts
  Constant26 : Constant  Value=zeros(2,1)  SampleTime=Model.PayloadMeas_sampling.Ts
  Constant27 : Constant  Value=zeros(3,1)  SampleTime=Model.MPS_sampling.Ts
  Demux1 : Demux  Outputs=3
  Demux10 : Demux  Outputs=3
  Demux9 : Demux  Outputs=3
  Discrete State-Space1 : DiscreteStateSpace  A=Kslew_opt_disc_zoh.A  B=Kslew_opt_disc_zoh.B  C=Kslew_opt_disc_zoh.C  D=Kslew_opt_disc_zoh.D  SampleTime=Model.ACS_sampling.Ts
  Gain : Gain  Gain=-1
  Mux2 : Mux  Inputs=6
  Sum : Sum  Inputs=+-
  Sum1 : Sum  Inputs=+-
  Sum2 : Sum  Inputs=+-
  Switch : Switch  Criteria=u2 > Threshold  ZeroCross=off
  Out1 : Outport  OutputWhenDisabled=reset  InitialOutput=0
  wires:
  Constant25/1 -> Bus Creator/5  "PMA_cmd"
  Demux9/1 -> Mux2/4
  Demux10/2 -> Sum1/2
  Demux9/3 -> Mux2/6
  Sum/1 -> Mux2/1
  Demux1/3 -> Sum2/1
  Gain/1 -> Demux9/1
  Demux10/3 -> Sum2/2
  Constant26/1 -> Bus Creator/4  "FSM_cmd"
  Demux1/1 -> Sum/1
  meas/1 -> Bus Selector1/1
  Constant27/1 -> Bus Creator/3  "MPS_cmd"
  Sum2/1 -> Mux2/3
  Sum1/1 -> Mux2/2
  Mux2/1 -> Discrete State-Space1/1
  Demux10/1 -> Sum/2
  Bus Selector1/1 -> Demux10/1  "<SST_meas>"
  ref/1 -> Demux1/1
  Constant/1 -> Bus Creator/1  "RW_cmd"
  Demux9/2 -> Mux2/5
  Demux1/2 -> Sum1/1
  Discrete State-Space1/1 -> Bus Creator/2  "RCS_cmd"
  Bus Selector1/2 -> Gain/1  "<GYRO_meas>"
  Bus Creator/1 -> Switch/1  "cmd"
  Constant21/1 -> Bus Creator2/4  "FSM_cmd"
  Constant24/1 -> Bus Creator2/1  "RW_cmd"
  Constant22/1 -> Bus Creator2/3  "MPS_cmd"
  Constant20/1 -> Bus Creator2/5  "PMA_cmd"
  Constant23/1 -> Bus Creator2/2  "RCS_cmd"
  Bus Creator2/1 -> Switch/3  "cmd"
  slew_deactivation/1 -> Switch/2
  Switch/1 -> Out1/1

== system Simscape_Benchmark_SIM1/Controllers/TransitionSlew2Coarse ==
  note: REMARK: Leave the name of the signals in the lines entering and exiting the "bus creator" block unaltered.
  note: This part can be modified by the user by selecting which strategy to implement for the switching between two controllers
  meas : Inport
  ref : Inport  Port=2
  Slew2CoarseActivation : Inport  Port=3
  Constant16 : Constant  Value=Model.ACS_sampling.Ts
  Slew 2 coarse switching : MATLAB Function  TreatAsAtomicUnit=on  SystemSampleTime=Model.ACS_sampling.Ts
  Slope : Constant  Value=0.25
  Subsystem : Subsystem
  Out1 : Outport  OutputWhenDisabled=reset  InitialOutput=0
  wires:
  ref/1 -> Subsystem/2(Input)
  Subsystem/1(cmd) -> Out1/1
  Slope/1 -> Slew 2 coarse switching/3(Slope)
  Slew2CoarseActivation/1 -> Slew 2 coarse switching/1(TransitionCoarse2FineActivation)
  Constant16/1 -> Slew 2 coarse switching/2(sampling)
  Slew 2 coarse switching/1(out1) -> Subsystem/3(out1)
  meas/1 -> Subsystem/1(In2)
  Slew 2 coarse switching/2(out2) -> Subsystem/4(out2)
